simulink model "bci_calibration_phase_research_system"  (R2013a)
settings: Solver=ode45  StartTime=0.0  StopTime=Inf  FixedStep=1  RelTol=1e-3
InitFcn:
  | clc % clear worskpace
  | clear all %clear all b=variables in workspace
model workspace (MAT data in the model file):
  local_ip = 2130706433
  local_port = 50224
  host_ip = 2130706433
  host_port = 50223
  serial_number = 'NB-2014.07.69'
  sample_rate = 250
  num_samples = 0
  num_en_channels = 32
  en_add_channels = 1
  cfg_native : struct (value not decoded)
undefined symbols (not defined in the file): NB
libraries: dspnetwork x2, simulink x1, gNautilusLib x1
settings Model: Creator=Yves Matanga  LastModifiedBy=Yves Matanga
settings SolverCC: ZeroCrossControl=EnableAll

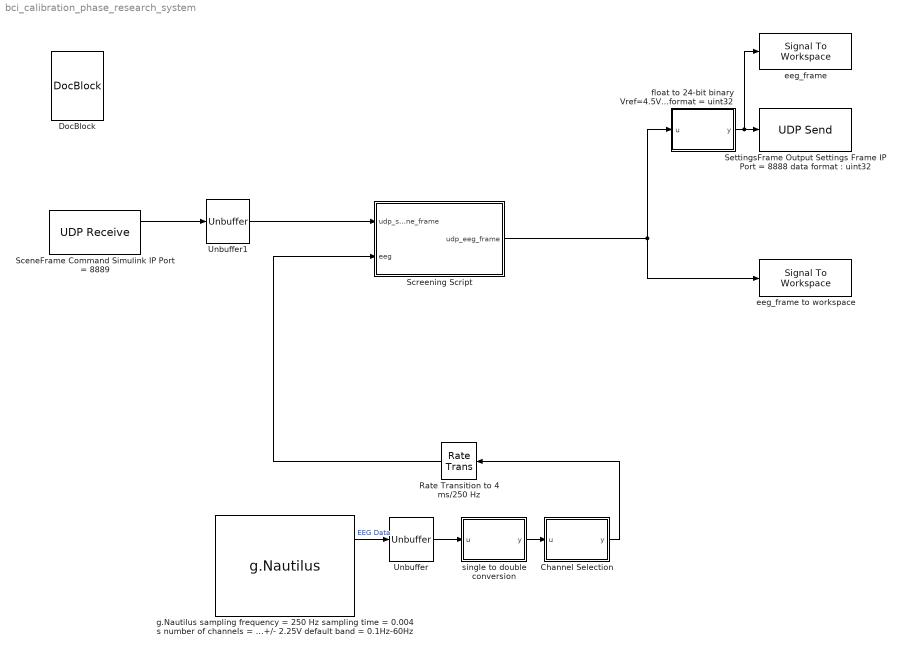
== system bci_calibration_phase_research_system ==
  Channel Selection : MATLAB Function  TreatAsAtomicUnit=on  SystemSampleTime=0.004
  DocBlock : simulink/Model-Wide Utilities/DocBlock  DocumentType=Text
      content=|
      | The Above platform is for EEG capturing a
      | and samping of screening imagery .
      |
      | A JAVA GUI is running aside this simulink and communicate
      | via UDP protocol
      |
      | Once the Screening start ,the Java scene GUI send a start
      | command to the simulink model (ASCII for '1' ) which
      | will trigger a sampling signal to 1
      |
      | Once the Screening stopped ,the Java GUI will send a stop command
      | to the simulink model (ASCII for '2') which will trigger
      | a sampling signal to 2
      |
      | else it iso 0
      |
      | the sampling signal will help extract the eeg signals of the
      | user motor imagery ,hence
      |
      | the interval between a start (1) and a stop (2) is
      | basically "a single trial eeg imagery"
      |
      | all the eeg signals will be transferred at all time to the java
      | application which save into a database for furhter recovery.
      |
      | Note that all blocks must have the sampling time as dictated by the EEG source
      | T = 0.004s (250Hz)
  Rate Transition to 4 ms/250 Hz : RateTransition  OutPortSampleTime=0.004
  SceneFrame Command Simulink IP Port = 8889 : dspnetwork/UDP Receive  localURL='0.0.0.0'  localPort=8889  remoteURL='127.0.0.1'  remotePort=-1  recvBufferSize=8192  dims=255  signalDatatype=uint8  isVarSize=off  showBlockingTime=off  blockingTime=0  sampletime=0.004
  Screening Script : MATLAB Function  TreatAsAtomicUnit=on  SystemSampleTime=0.004
  "SettingsFrame Output Settings Frame IP Port = 8888 data format : uint32" : dspnetwork/UDP Send  remoteURL='127.0.0.1'  remotePort=8888  localURL='0.0.0.0'  localPortSource=Automatically determine  localPort=-1  sampletime=-1  separateLengthPort=0
  Unbuffer : Unbuffer  SampleBasedProcessing=Same as frame based
  Unbuffer1 : Unbuffer  SampleBasedProcessing=Same as frame based
  eeg_frame : SignalToWorkspace  VariableName=digitized_eeg_frame
      settings: CopyFcn=dspblkcopystw(gcbh);
  eeg_frame to workspace : SignalToWorkspace  VariableName=eeg_frame
      settings: CopyFcn=dspblkcopystw(gcbh);
  float to 24-bit binary Vref=4.5V(in uV) Mean = 2.25V data format = uint32 : MATLAB Function  TreatAsAtomicUnit=on  SystemSampleTime=0.004
  "g.Nautilus sampling frequency = 250 Hz sampling time = 0.004 s number of channels = 32 resolution = 24 Bit output = float32 unit = uV dynamic range = +/- 2.25V default band = 0.1Hz-60Hz " : gNautilusLib/g.Nautilus  Tag=g.Nautilus  Description=Operates a g.Nautilus device and provides acquired data on its outputs.  sample_rate=250  local_ip=2130706433  local_port=50224  host_ip=2130706433  host_port=50223  serial_number=NB-2014.07.69  num_samples=0  num_en_channels=32  add_channels=1
  single to double conversion : MATLAB Function  TreatAsAtomicUnit=on  SystemSampleTime=0.004
  wires:
  "g.Nautilus sampling frequency = 250 Hz sampling time = 0.004 s number of channels = 32 resolution = 24 Bit output = float32 unit = uV dynamic range = +/- 2.25V default band = 0.1Hz-60Hz "/1 -> Unbuffer/1  "EEG Data"
  Unbuffer/1 -> single to double conversion/1(u)
  single to double conversion/1(y) -> Channel Selection/1(u)
  Unbuffer1/1 -> Screening Script/1(udp_scene_frame)
  SceneFrame Command Simulink IP Port = 8889/1 -> Unbuffer1/1
  Screening Script/1(udp_eeg_frame) -> eeg_frame to workspace/1, float to 24-bit binary Vref=4.5V(in uV) Mean = 2.25V data format = uint32/1(u)
  Channel Selection/1(y) -> Rate Transition to 4 ms/250 Hz/1
  Rate Transition to 4 ms/250 Hz/1 -> Screening Script/2(eeg)
  float to 24-bit binary Vref=4.5V(in uV) Mean = 2.25V data format = uint32/1(y) -> eeg_frame/1, "SettingsFrame Output Settings Frame IP Port = 8888 data format : uint32"/1

== matlab function bci_calibration_phase_research_system/single to double conversion ==
  data: u input; y output
function y = fcn(u)
%#codegen
y = double(u);

== matlab function bci_calibration_phase_research_system/Screening Script ==
  data: udp_scene_frame input; eeg input; udp_eeg_frame output
function udp_eeg_frame  = fcn( udp_scene_frame,eeg)
%#codegen
 if udp_scene_frame == uint8('1') %START in ASCII
     udp_eeg_frame = [eeg 1];%timing frame = 1
 elseif udp_scene_frame == uint8('2') %STOP
     udp_eeg_frame = [eeg 2];%timing frame = 2
 else
     udp_eeg_frame = [eeg 0];%timing frame = 0
 end
 
 %the purpose of this function to 
 %save the  eeg signals sampled with the start
 %and stop of every trial%

== matlab function bci_calibration_phase_research_system/Channel Selection ==
  data: u input; y output
function y = fcn(u)
%#codegen

%channel lookup table
% 1 --  FP1                      % 17 --  C4
% 2 --  FP2                      % 18 --  T8
% 3 --  AF3                      % 19 --  CP5
% 4 --  AF4                      % 20 --  CP1
% 5 --  F7                       % 21 --  CP2
% 6 --  F3                       % 22 --  CP6
% 7 --  FZ                       % 23 --  P7 
% 8 --  F4                       % 24 --  P3
% 9 --  F8                       % 25 --  PZ
% 10 -- FC5                      % 26 --  P4
% 11 -- FC1                      % 27 --  P8
% 12 -- FC2                      % 28 --  PO7
% 13 -- FC6                      % 29 --  PO3
% 14 -- T7                       % 30 --  PO4
% 15 -- C3                       % 31 --  PO8
% 16 -- CZ                       % 32 --  OZ

y = [u]; %Select All Channels

== matlab function bci_calibration_phase_research_system/float to 24-bit binary Vref=4.5V(in uV) Mean = 2.25V data format = uint32 ==
  data: u input; y output
function y = fcn(u)
 eeg_frame = u(1:32);
 %convert to 24 bit binary
 bin = uint32((eeg_frame + 2.25e6)*(2^24-1)/(4.5e6));
y = [bin uint32(u(33))]; %Select All Channels
